simulink model "approxctrlsim"  (Simulink 7.1)
settings: Solver=ode1  StartTime=0.0  StopTime=10.0  FixedStep=0.1/f  RelTol=1e-3
values from neighbouring files (symbols this model uses):
  f = handles.f    [aliasing.m]    (also in approx.m = fvec(i); approxctrl.m = fvec(i); approxctrl2.m = fvec(i); boded.m = fvec(i))
libraries: cstblocks x4
settings Model: Creator=rpm  LastModifiedBy=rpm
settings DataIOCC: LimitDataPoints=off  SaveOutput=off  SignalLogging=off  TimeSaveName=td

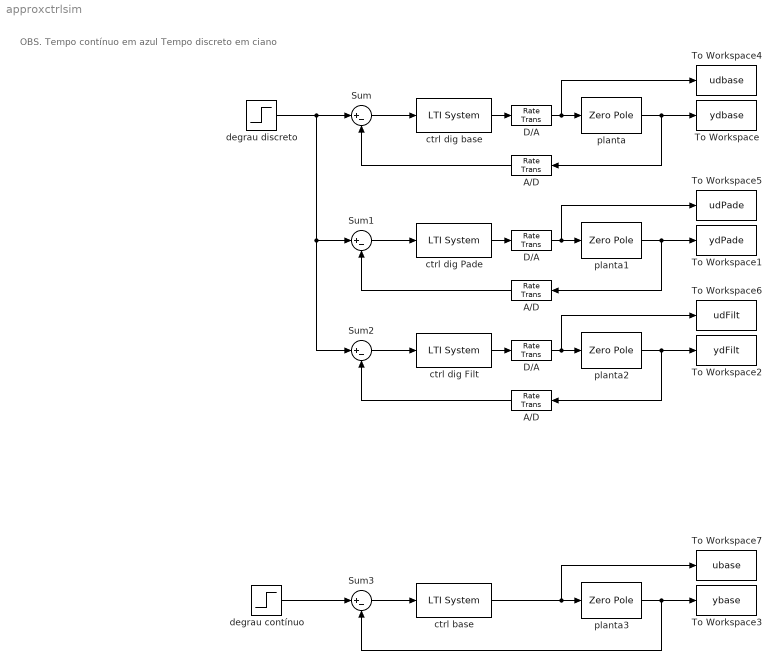
== system approxctrlsim ==
  note: OBS.
      | Tempo contínuo em azul
      | Tempo discreto em ciano
  "  A/D  " : RateTransition  Orientation=left  OutPortSampleTime=1/f
  "  D/A  " : RateTransition  Integrity=off  OutPortSampleTimeOpt=Inherit
  " A/D " : RateTransition  Orientation=left  OutPortSampleTime=1/f
  " D/A " : RateTransition  Integrity=off  Deterministic=off  OutPortSampleTimeOpt=Inherit
  A/D : RateTransition  Orientation=left  OutPortSampleTime=1/f
  D/A : RateTransition  Integrity=off  Deterministic=off  OutPortSampleTimeOpt=Inherit  OutPortSampleTime=0
  Sum : Sum  Inputs=|+-  OutDataType=sfix(16)  OutScaling=2^0  SampleTime=1/f
  Sum1 : Sum  Inputs=|+-  OutDataType=sfix(16)  OutScaling=2^0  SampleTime=1/f
  Sum2 : Sum  Inputs=|+-  OutDataType=sfix(16)  OutScaling=2^0  SampleTime=1/f
  Sum3 : Sum  Inputs=|+-  OutDataType=sfix(16)  OutScaling=2^0
  To Workspace : ToWorkspace  VariableName=ydbase  SampleTime=-1  SaveFormat=Structure
  To Workspace1 : ToWorkspace  VariableName=ydPade  SampleTime=-1  SaveFormat=Structure
  To Workspace2 : ToWorkspace  VariableName=ydFilt  SampleTime=-1  SaveFormat=Structure
  To Workspace3 : ToWorkspace  VariableName=ybase  SampleTime=-1  SaveFormat=Structure
  To Workspace4 : ToWorkspace  VariableName=udbase  SampleTime=-1  SaveFormat=Structure
  To Workspace5 : ToWorkspace  VariableName=udPade  SampleTime=-1  SaveFormat=Structure
  To Workspace6 : ToWorkspace  VariableName=udFilt  SampleTime=-1  SaveFormat=Structure
  To Workspace7 : ToWorkspace  VariableName=ubase  SampleTime=-1  SaveFormat=Structure
  ctrl base : cstblocks/LTI System  SystemSampleTime=-1  sys=ctrlbase  IC=[]
  ctrl dig Filt : cstblocks/LTI System  SystemSampleTime=-1  sys=ctrldFilt  IC=[]
  ctrl dig Pade : cstblocks/LTI System  SystemSampleTime=-1  sys=ctrldPade  IC=[]
  ctrl dig base : cstblocks/LTI System  SystemSampleTime=-1  sys=ctrldbase  IC=[]
  degrau contínuo : Step  Time=0  SampleTime=0
  degrau discreto : Step  Time=0  SampleTime=1/f
  planta{,1..3} (4 alike) : ZeroPole  Zeros=[]  Poles=[0 -1]
  wires:
  ctrl dig base/1 -> D/A/1
  Sum/1 -> ctrl dig base/1
  planta/1 -> To Workspace/1, A/D/1
  ctrl dig Pade/1 -> " D/A "/1
  Sum1/1 -> ctrl dig Pade/1
  planta1/1 -> To Workspace1/1, " A/D "/1
  ctrl dig Filt/1 -> "  D/A  "/1
  Sum2/1 -> ctrl dig Filt/1
  planta2/1 -> To Workspace2/1, "  A/D  "/1
  degrau discreto/1 -> Sum/1, Sum1/1, Sum2/1
  A/D/1 -> Sum/2
  " A/D "/1 -> Sum1/2
  "  A/D  "/1 -> Sum2/2
  D/A/1 -> planta/1, To Workspace4/1
  " D/A "/1 -> planta1/1, To Workspace5/1
  "  D/A  "/1 -> planta2/1, To Workspace6/1
  degrau contínuo/1 -> Sum3/1
  Sum3/1 -> ctrl base/1
  ctrl base/1 -> planta3/1, To Workspace7/1
  planta3/1 -> To Workspace3/1, Sum3/2
